simulink model "FinalProject_EE547_Step14"  (R2018b)
settings: Solver=VariableStepAuto  StartTime=0.0  StopTime=10.0  RelTol=1e-3
values from neighbouring files (symbols this model uses):
  C = eye(4)    [Goniodsky_Mistry_EE547_ProjectCode.m]
  D = zeros(4,1)    [Goniodsky_Mistry_EE547_ProjectCode.m]
  K = place(A,B,poles1)    [Goniodsky_Mistry_EE547_ProjectCode.m]
undefined symbols (not defined in the file or in its folder): A, B
settings Model: Creator=GAJJAR  LastModifiedBy=GAJJAR

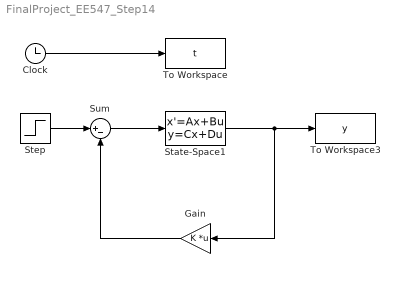
== system FinalProject_EE547_Step14 ==
  Clock : Clock
  Gain : Gain  Gain=K  Multiplication=Matrix(K*u)
  State-Space1 : StateSpace  A=A  B=B  C=C  D=D  InitialCondition=0
  Step : Step  Time=0  SampleTime=0
  Sum : Sum  Inputs=|+-
  To Workspace : ToWorkspace  VariableName=t  SampleTime=-1
  To Workspace3 : ToWorkspace  VariableName=y  SampleTime=-1
  wires:
  State-Space1/1 -> Gain/1, To Workspace3/1
  Clock/1 -> To Workspace/1
  Step/1 -> Sum/1
  Gain/1 -> Sum/2
  Sum/1 -> State-Space1/1
